simulink model "Exercicio_6_Vinicius_2"  (R2015a)
settings: Solver=ode45  StartTime=0.0  StopTime=3  FixedStep=Ts  RelTol=1e-3
undefined symbols (not defined in the file): AA, BB, DD, E, F, H, Ts, W
libraries: cstblocks x1
settings Model: Creator=vinic  LastModifiedBy=vinic

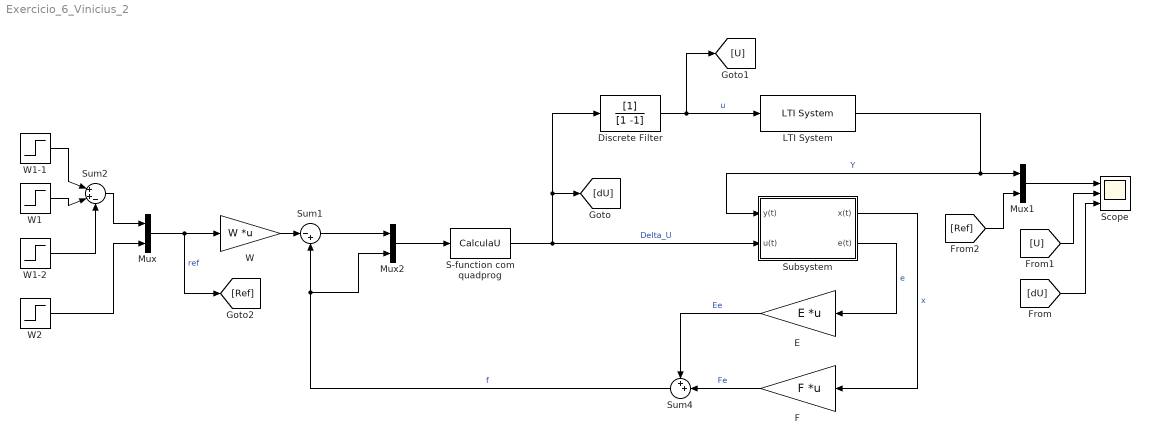
== system Exercicio_6_Vinicius_2 ==
  Discrete Filter : DiscreteFilter  Denominator=[1 -1]  SampleTime=Ts
  E : Gain  Gain=E  Multiplication=Matrix(K*u)
  F : Gain  Gain=F  Multiplication=Matrix(K*u)
  LTI System : cstblocks/LTI System  sys=Ct  IC=[]
  Mux : Mux  Inputs=2
  Mux1 : Mux  Inputs=2
  Mux2 : Mux  Inputs=2
  S-function com quadprog : S-Function  FunctionName=CalculaU  Parameters=Parametros
  Scope : Scope  NumInputPorts=3
      settings: YMin=0~2.77556e-17~-0.2  YMax=0.8~0.8~0.8  SaveName=simul
  Subsystem : Subsystem
  Sum1 : Sum  Inputs=|-+
  Sum2 : Sum  Inputs=|++-
  Sum4 : Sum  Inputs=++|
  W : Gain  Gain=W  Multiplication=Matrix(K*u)
  W1 : Step  Time=0  After=0.4  SampleTime=Ts
  W1-1 : Step  Time=2  After=0.3  SampleTime=Ts
  W1-2 : Step  After=0.1  SampleTime=Ts
  W2 : Step  Time=0  After=0.2  SampleTime=Ts
  wires:
  LTI System/1 -> Mux1/1, Subsystem/1(y(t))  "Y"
  Mux/1 -> [Ref], W/1  "ref"
  W2/1 -> Mux/2
  Sum2/1 -> Mux/1
  Mux1/1 -> Scope/1
  Discrete Filter/1 -> LTI System/1, [U]  "u"
  Sum4/1 -> Sum1/2, Mux2/2  "f"
  W/1 -> Sum1/1
  S-function com quadprog/1 -> [dU], Discrete Filter/1, Subsystem/2(u(t))  "Delta_U"
  Mux2/1 -> S-function com quadprog/1
  Sum1/1 -> Mux2/1
  Subsystem/1(x(t)) -> F/1  "x"
  Subsystem/2(e(t)) -> E/1  "e"
  F/1 -> Sum4/2  "Fe"
  E/1 -> Sum4/1  "Ee"
  [dU] -> Scope/3
  [U] -> Scope/2
  [Ref] -> Mux1/2
  W1/1 -> Sum2/2
  W1-2/1 -> Sum2/3
  W1-1/1 -> Sum2/1

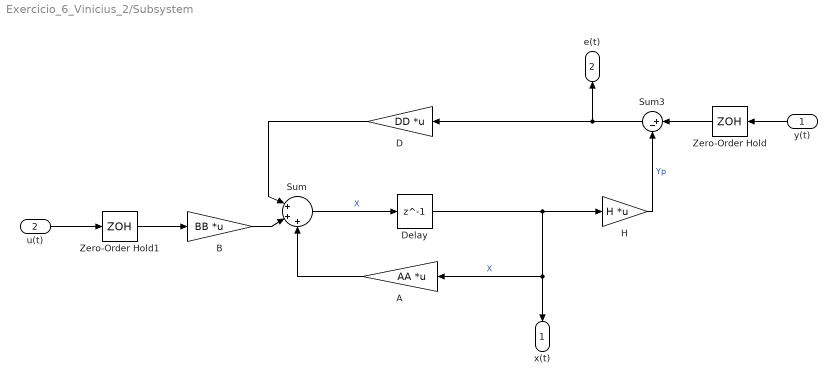
== system Exercicio_6_Vinicius_2/Subsystem ==
  y(t) : Inport
  u(t) : Inport  Port=2
  A : Gain  Gain=AA  Multiplication=Matrix(K*u)
  B : Gain  Gain=BB  Multiplication=Matrix(K*u)
  D : Gain  Gain=DD  Multiplication=Matrix(K*u)
  Delay : Delay  DelayLength=1  SampleTime=Ts
  H : Gain  Gain=H  Multiplication=Matrix(K*u)
  Sum : Sum  Inputs=|+++
  Sum3 : Sum  Inputs=|+-
  Zero-Order Hold : ZeroOrderHold  SampleTime=Ts
  Zero-Order Hold1 : ZeroOrderHold  SampleTime=Ts
  x(t) : Outport
  e(t) : Outport  Port=2
  wires:
  y(t)/1 -> Zero-Order Hold/1
  u(t)/1 -> Zero-Order Hold1/1
  A/1 -> Sum/3
  B/1 -> Sum/2
  D/1 -> Sum/1
  Delay/1 -> x(t)/1, A/1, H/1  "X"
  Sum/1 -> Delay/1  "X"
  Zero-Order Hold1/1 -> B/1
  Zero-Order Hold/1 -> Sum3/1
  H/1 -> Sum3/2  "Yp"
  Sum3/1 -> D/1, e(t)/1
